simulink model "simulink_eolienne"  (R2019b)
settings: Solver=VariableStepAuto  StartTime=0.0  StopTime=170  RelTol=1e-3
values from neighbouring files (symbols this model uses):
  A = [1.5 0 0 0; 0 3 0 0; 0 0 0.5 0; 0 0 0 0.9]    [BE1.m]    (also in BE2a5.m = [a 0 ; (3*alpha0*v0^2)/(J*w0) (-alpha0*v0^3)/(J*w0^2)])
  C = [1 1 1 0; 0 1 3 1]    [BE1.m]    (also in BE2a5.m = [0  1])
  F = inv(R + B'*P*B)*B'*P*A    [BE1.m]
  K = lqr(A',C',W,V)'    [BE2a5.m]
  x0 = [2 2 2 2]'    [BE1.m]
undefined symbols (not defined in the file or in its folder): BE, Ce, Fplus, H, x0bis
settings Model: Creator=wasselia  LastModifiedBy=antoi
settings DataIOCC: ReturnWorkspaceOutputs=off
settings DebuggingCC: ArithmeticOperatorsInVariantConditions=warning
settings SFSimCC: CustomCodeUndefinedFunction=UseInterfaceOnly

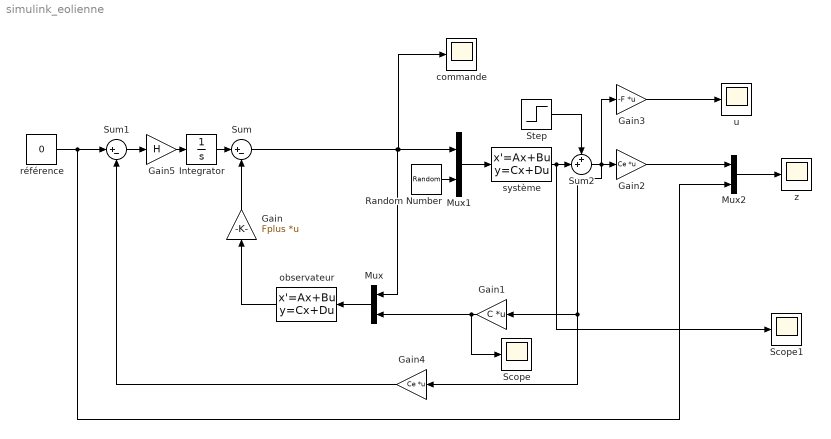
== system simulink_eolienne ==
  Gain : Gain  Gain=Fplus  Multiplication=Matrix(K*u)
  Gain1 : Gain  Gain=C  Multiplication=Matrix(K*u) (u vector)
  Gain2 : Gain  Gain=Ce  Multiplication=Matrix(K*u) (u vector)
  Gain3 : Gain  Gain=-F  Multiplication=Matrix(K*u) (u vector)
  Gain4 : Gain  Gain=Ce  Multiplication=Matrix(K*u) (u vector)
  Gain5 : Gain  Gain=H
  Integrator : Integrator
  Mux : Mux  Inputs=2
  Mux1 : Mux  Inputs=2
  Mux2 : Mux  Inputs=2
  Random Number : RandomNumber  Mean=0.5  Variance=0.01  SampleTime=1
  Scope : Scope
  Scope1 : Scope
  Step : Step  Time=100  SampleTime=0
  Sum : Sum  Inputs=|+-
  Sum1 : Sum  Inputs=|+-
  Sum2 : Sum  Inputs=++|
  commande : Scope
  observateur : StateSpace  A=A-K*C  B=BE  C=[1 0;0 1]  D=[0 0 ; 0 0]  InitialCondition=x0
  référence : Constant  Value=0
  système : StateSpace  A=A  B=BE  C=[1 0;0 1]  D=[0 0 ; 0 0]  InitialCondition=x0bis
  u : Scope
  z : Scope
  wires:
  Mux/1 -> observateur/1
  Gain/1 -> Sum/2
  Mux1/1 -> système/1
  Random Number/1 -> Mux1/2
  Sum/1 -> Mux/1, commande/1, Mux1/1
  Gain3/1 -> u/1
  Gain1/1 -> Scope/1, Mux/2
  système/1 -> Scope1/1, Sum2/2
  Sum2/1 -> Gain3/1, Gain4/1, Gain1/1, Gain2/1
  Step/1 -> Sum2/1
  référence/1 -> Mux2/2, Sum1/1
  Gain4/1 -> Sum1/2
  Integrator/1 -> Sum/1
  Gain5/1 -> Integrator/1
  Sum1/1 -> Gain5/1
  Mux2/1 -> z/1
  Gain2/1 -> Mux2/1
  observateur/1 -> Gain/1
